simulink model "TEME_2_ECI_test"  (R2016b)
settings: Solver=VariableStepAuto  StartTime=0.0  StopTime=1  RelTol=1e-3
values from neighbouring files (symbols this model uses):
  JD = JD_ut1(1)    [coord_rot_time_test_init.m]
  JD_2_cent = 1/(36525)    (= 2.73785078713e-05)    [coord_rot_time_test_init.m]
  rTEME = [ -9060.47373569; 4658.70952502; 813.68673153 ]    [coord_rot_time_test_init.m]
  sec_2_cent = 1/(86400*36525)    (= 3.1688087814e-10)    [coord_rot_time_test_init.m]
  ut1_2_tt = 32.184 + 32 + dut1    (= 64.388241)    [coord_rot_time_test_init.m]
  vTEME = [ -2.232832783; -4.110453490; -3.157345433 ]    [coord_rot_time_test_init.m]
libraries: coord_rotation_lib x1
settings Model: Creator=taylorreynolds  LastModifiedBy=taylorreynolds

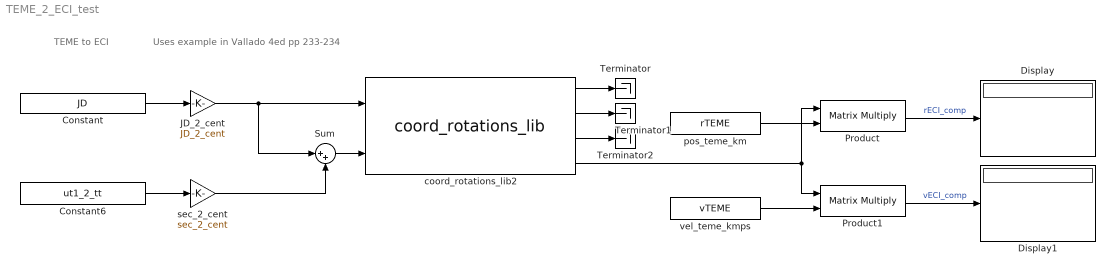
== system TEME_2_ECI_test ==
  note: Uses example in Vallado 4ed pp 233-234
  note: TEME to ECI
  Constant : Constant  Value=JD
  Constant6 : Constant  Value=ut1_2_tt
  Display : Display
  Display1 : Display
  JD_2_cent : Gain  Gain=JD_2_cent
  Product : Product  Multiplication=Matrix(*)
  Product1 : Product  Multiplication=Matrix(*)
  Sum : Sum  Inputs=|++
  Terminator : Terminator
  Terminator1 : Terminator
  Terminator2 : Terminator
  coord_rotations_lib2 : coord_rotation_lib/coord_rotations_lib
  pos_teme_km : Constant  Value=rTEME
  sec_2_cent : Gain  Gain=sec_2_cent
  vel_teme_kmps : Constant  Value=vTEME
  wires:
  Constant/1 -> JD_2_cent/1
  JD_2_cent/1 -> coord_rotations_lib2/1, Sum/1
  sec_2_cent/1 -> Sum/2
  Sum/1 -> coord_rotations_lib2/2
  coord_rotations_lib2/1 -> Terminator/1
  coord_rotations_lib2/3 -> Terminator2/1
  coord_rotations_lib2/2 -> Terminator1/1
  coord_rotations_lib2/4 -> Product/1, Product1/1
  pos_teme_km/1 -> Product/2
  vel_teme_kmps/1 -> Product1/2
  Product/1 -> Display/1  "rECI_comp"
  Product1/1 -> Display1/1  "vECI_comp"
  Constant6/1 -> sec_2_cent/1
